simulink model "CounterUpDown_RE_test_harness"  (R2013a)
settings: Solver=ode3  StartTime=0.0  StopTime=10  RelTol=1e-3
undefined symbols (not defined in the file): sigbuilder_block
libraries: simulink x1
settings Model: SldvGeneratedHarnessModel=TestUnitModel=CounterUpDown_RE_test|  CovMetricSettings=dcmoe  CovHTMLOptions=-aTS=1 -bRG=1 -bTC=0 -hTR=0 -nFC=0 -scm=1 -bcm=1  CovModelRefEnable=on  CovExternalEMLEnable=on  Creator=kyle.willis  LastModifiedBy=kyle.willis
settings DataIOCC: SaveFormat=StructureWithTime  ReturnWorkspaceOutputs=on
settings OptimizationCC: InlineParams=on
settings DebuggingCC: InheritedTsInSrcMsg=none

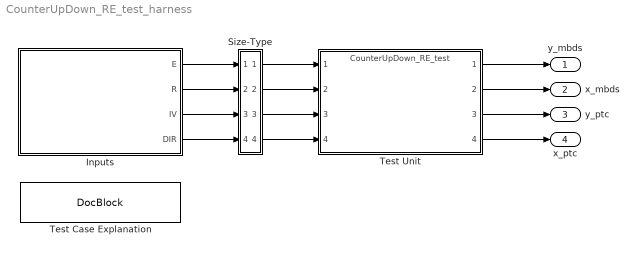
== system CounterUpDown_RE_test_harness ==
  Inputs : Subsystem  Tag=STV Subsys  LoadFcn=sigbuilder_block('load',[480.75 176.25 519.75 395.25 ]);  StartFcn=sigbuilder_block('start');  StopFcn=sigbuilder_block('stop');  ClipboardFcn=sigbuilder_block('clipboard');  mask(Sigbuilder block){}
      mask init:
      | if ~strcmp(get_param(bdroot(gcb),'SimulationStatus'),'stopped'),tuvar = sigbuilder_block('maskInit'); end
      settings: CopyFcn=sigbuilder_block('copy');  DeleteFcn=sigbuilder_block('delete');  ModelCloseFcn=sigbuilder_block('modelClose');  PreSaveFcn=sigbuilder_block('preSave');  PauseFcn=sigbuilder_block('pause');  ContinueFcn=sigbuilder_block('continue');  NameChangeFcn=sigbuilder_block('namechange');  OpenFcn=sigbuilder_block('open');  CloseFcn=sigbuilder_block('close');
      mask Display: plot(0, 0, 100, 100,[2, 2, 32, 32, 2], [68, 8, 8, 68, 68],[32, 2], [38, 38], [32, 19, 2],[53, 60, 44], [32, 17, 17, 2],[16, 16, 31, 31]);txt = getActiveGroup(gcbh);text(2, 100, txt,'verticalAlignment', 'top');
  Size-Type : Subsystem
  Test Case Explanation : simulink/Model-Wide Utilities/DocBlock  DocumentType=Text
  Test Unit : ModelReference  ModelNameDialog=CounterUpDown_RE_test  SimulationMode=Normal  ModelReferenceVersion=1.6  CopyOfModelName=CounterUpDown_RE_test  DefaultDataLogging=on
  y_mbds : Outport
  x_mbds : Outport  Port=2
  y_ptc : Outport  Port=3
  x_ptc : Outport  Port=4
  wires:
  Size-Type/1(Out1) -> Test Unit/1
  Size-Type/2(Out2) -> Test Unit/2
  Size-Type/3(Out3) -> Test Unit/3
  Size-Type/4(Out4) -> Test Unit/4
  Test Unit/1 -> y_mbds/1
  Test Unit/2 -> x_mbds/1
  Test Unit/3 -> y_ptc/1
  Test Unit/4 -> x_ptc/1
  Inputs/1(E) -> Size-Type/1(In1)
  Inputs/4(DIR) -> Size-Type/4(In4)
  Inputs/2(R) -> Size-Type/2(In2)
  Inputs/3(IV) -> Size-Type/3(In3)

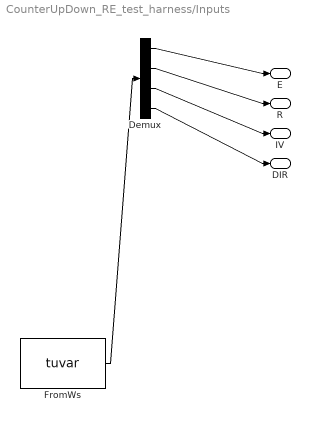
== system CounterUpDown_RE_test_harness/Inputs ==
  Demux : Demux  Tag=STV Demux
  FromWs : FromWorkspace  Tag=STV FromWs  VariableName=tuvar  SampleTime=0
      SigBuilderData=|
      | dataSet(1).timeRange = [0 0.032]
      | dataSet(1).name = 'Sheet1'
      | dataSet(2).timeRange = [0 0.032]
      | dataSet(2).name = 'Sheet2'
      | sbobj.Name = 'Signal Builder'
      | sbobj.Groups(1).Name = 'Sheet1'
      | sbobj.Groups(1).Signals(1).Name = 'E'
      | sbobj.Groups(1).Signals(1).XData = [0 0.001 0.002 0.003 0.004 0.005 0.006 0.007 0.008 0.009 0.01 0.011 0.012 0.013 0.014 0.015 0.016 0.017 0.018 0.019 0.02 0.021 0.022 0.023 0.024 0.025 0.026 0.027 0.028 0.029 0.03 0.031 0.032]
      | sbobj.Groups(1).Signals(1).YData = [0 0 0 0 1 1 1 1 0 0 0 0 1 1 1 1 0 0 0 0 1 1 1 1 0 0 0 0 1 1 1 1 0]
      | sbobj.Groups(1).Signals(2).Name = 'R'
      | sbobj.Groups(1).Signals(2).XData = [0 0.001 0.002 0.003 0.004 0.005 0.006 0.007 0.008 0.009 0.01 0.011 0.012 0.013 0.014 0.015 0.016 0.017 0.018 0.019 0.02 0.021 0.022 0.023 0.024 0.025 0.026 0.027 0.028 0.029 0.03 0.031 0.032]
      | sbobj.Groups(1).Signals(2).YData = [0 0 1 1 0 0 1 1 0 0 1 1 0 0 1 1 0 0 1 1 0 0 1 1 0 0 1 1 0 0 1 1 0]
      | sbobj.Groups(1).Signals(3).Name = 'IV'
      | sbobj.Groups(1).Signals(3).XData = [0 0.001 0.002 0.003 0.004 0.005 0.006 0.007 0.008 0.009 0.01 0.011 0.012 0.013 0.014 0.015 0.016 0.017 0.018 0.019 0.02 0.021 0.022 0.023 0.024 0.025 0.026 0.027 0.028 0.029 0.03 0.031 0.032]
      | sbobj.Groups(1).Signals(3).YData = [0 1 0 1 0 1 0 1 0 1 0 1 0 1 0 1 0 1 0 1 0 1 0 1 0 1 0 1 0 1 0 1 0]
      | sbobj.Groups(1).Signals(4).Name = 'DIR'
      | sbobj.Groups(1).Signals(4).XData = [0 0.001 0.002 0.003 0.004 0.005 0.006 0.007 0.008 0.009 0.01 0.011 0.012 0.013 0.014 0.015 0.016 0.017 0.018 0.019 0.02 0.021 0.022 0.023 0.024 0.025 0.026 0.027 0.028 0.029 0.03 0.031 0.032]
      | sbobj.Groups(1).Signals(4).YData = [0 0 0 0 0 0 0 0 1 1 1 1 1 1 1 1 1 1 0 1 0 0 0 0 0 1 0 1 1 0 1 1 1]
      | sbobj.Groups(1).TimeRange = [0 0.032]
      | sbobj.Groups(2).Name = 'Sheet2'
      | sbobj.Groups(2).Signals(1).Name = 'E'
      | sbobj.Groups(2).Signals(1).XData = [0 0.001 0.002 0.003 0.004 0.005 0.006 0.007 0.008 0.009 0.01 0.011 0.012 0.013 0.014 0.015 0.016 0.017 0.018 0.019 0.02 0.021 0.022 0.023 0.024 0.025 0.026 0.027 0.028 0.029 0.03 0.031 0.032]
      | sbobj.Groups(2).Signals(1).YData = [89513 -15001 91966 45155 86440 62225 95463 92340 78142 88665 -64008 -62432 59186 106 55794 -17437 8614 81848 -52243 16773 -51986 -26514 16008 -88528 52713 55072 16673 -25581 69300 50367 -70604 -32261 84192]
      | sbobj.Groups(2).Signals(2).Name = 'R'
      | sbobj.Groups(2).Signals(2).XData = [0 0.001 0.002 0.003 0.004 0.005 0.006 0.007 0.008 0.009 0.01 0.011 0.012 0.013 0.014 0.015 0.016 0.017 0.018 0.019 0.02 0.021 0.022 0.023 0.024 0.025 0.026 0.027 0.028 0.029 0.03 0.031 0.032]
      | sbobj.Groups(2).Signals(2).YData = [-5486 90656 18797 70279 -46004 48739 14869 4812 26542 -55942 53507 25739 58960 -90019 -83654 -37875 -98399 22694 -53851 30884 21261 -17729 -16594 -80405 -46734 -21103 38384 -1249 21681 62663 -93195 -11235 -9373]
      | sbobj.Groups(2).Signals(3).Name = 'IV'
      | sbobj.Groups(2).Signals(3).XData = [0 0.001 0.002 0.003 0.004 0.005 0.006 0.007 0.008 0.009 0.01 0.011 0.012 0.013 0.014 0.015 0.016 0.017 0.018 0.019 0.02 0.021 0.022 0.023 0.024 0.025 0.026 0.027 0.028 0.029 0.03 0.031 0.032]
      | sbobj.Groups(2).Signals(3).YData = [-73240 9821 -67618 88555 -2879 -56471 94063 -36268 -42818 -76871 8537 82097 -63122 20812 -66209 -50721 -50608 85723 61916 20597 -83847 11433 -63223 92421 46966 -37181 30197 -80267 6278 79991 5339 4970 33718]
      | sbobj.Groups(2).Signals(4).Name = 'DIR'
      | sbobj.Groups(2).Signals(4).XData = [0 0.001 0.002 0.003 0.004 0.005 0.006 0.007 0.008 0.009 0.01 0.011 0.012 0.013 0.014 0.015 0.016 0.017 0.018 0.019 0.02 0.021 0.022 0.023 0.024 0.025 0.026 0.027 0.028 0.029 0.03 0.031 0.032]
      | sbobj.Groups(2).Signals(4).YData = [1 1 1 0 0 0 0 1 1 0 1 1 1 0 0 1 1 -31029 88069 -69590 -68727 65912 -9360 68634 -60667 44155 13182 -1453 -48555 -14278 -31220 38977 -88052]
      | sbobj.Groups(2).TimeRange = [0 0.032]
  E : Outport
  R : Outport  Tag=STV Outport  Port=2
  IV : Outport  Tag=STV Outport  Port=3
  DIR : Outport  Tag=STV Outport  Port=4
  wires:
  FromWs/1 -> Demux/1
  Demux/1 -> E/1
  Demux/2 -> R/1
  Demux/3 -> IV/1
  Demux/4 -> DIR/1

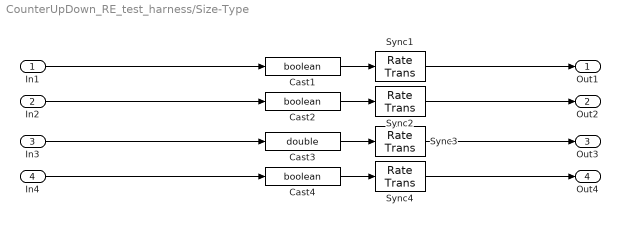
== system CounterUpDown_RE_test_harness/Size-Type ==
  In1 : Inport
  In2 : Inport  Port=2
  In3 : Inport  Port=3
  In4 : Inport  Port=4
  Cast1 : DataTypeConversion  OutDataTypeStr=boolean  SaturateOnIntegerOverflow=on  RndMeth=Zero
  Cast2 : DataTypeConversion  OutDataTypeStr=boolean  SaturateOnIntegerOverflow=on  RndMeth=Zero
  Cast3 : DataTypeConversion  OutDataTypeStr=double  SaturateOnIntegerOverflow=on  RndMeth=Zero
  Cast4 : DataTypeConversion  OutDataTypeStr=boolean  SaturateOnIntegerOverflow=on  RndMeth=Zero
  Sync{1..4} (4 alike) : RateTransition  OutPortSampleTime=[0.20000000000000001,0]
  Out1 : Outport
  Out2 : Outport  Port=2
  Out3 : Outport  Port=3
  Out4 : Outport  Port=4
  wires:
  In1/1 -> Cast1/1
  Cast1/1 -> Sync1/1
  Sync1/1 -> Out1/1
  In2/1 -> Cast2/1
  Cast2/1 -> Sync2/1
  Sync2/1 -> Out2/1
  In3/1 -> Cast3/1
  Cast3/1 -> Sync3/1
  Sync3/1 -> Out3/1
  In4/1 -> Cast4/1
  Cast4/1 -> Sync4/1
  Sync4/1 -> Out4/1
